simulink model "Outer1"  (Simulink 5.0)
settings: Solver=ode45  StartTime=0.0  StopTime=10.0  RelTol=1e-3
settings Model: Creator=scaife  LastModifiedBy=scaife  ExtModeAutoUpdateStatusClock=off

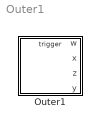
== system Outer1 ==
  Outer1 : Stateflow chart

== stateflow chart Outer1 ==
  state A/
    en: z++;
    ex: w++;
  (default) -> A
  A -> A : E{x++;}/y++;
  data: w output int32; x output int32; z output int32; y output int32
  events: E input EITHER_EDGE_EVENT
